simulink model "orangery_next_generation"  (R2020b)
settings: Solver=ode45  StartTime=86000*600  StopTime=86000*607  FixedStep=0.01  MaxStep=1  RelTol=1e-6  EnableMultiTasking=on
settings Model: Creator=oleg.kmechak  LastModifiedBy=ofcra
settings DataIOCC: LimitDataPoints=on  SaveFinalState=on  SaveFormat=Array  ReturnWorkspaceOutputs=off
settings OptimizationCC: LifeSpan=inf
settings DebuggingCC: UnderspecifiedInitializationDetection=Classic  MergeDetectMultiDrivingBlocksExec=none  SolverPrmCheckMsg=warning  SFUnexpectedBacktrackingDiag=warning  SFNoUnconditionalDefaultTransitionDiag=warning  SFExecutionAtInitializationDiag=none  ArithmeticOperatorsInVariantConditions=warning
settings HardwareCC: ProdBitPerPointer=32  ProdBitPerSizeT=32  ProdBitPerPtrDiffT=32  ProdLargestAtomicFloat=None  ProdIntDivRoundTo=Undefined  ProdEndianess=Unspecified  ProdWordSize=32  ProdHWDeviceType=32-bit Generic
settings ModelReferenceCC: PropagateSignalLabelsOutOfModel=off
settings SFSimCC: SimUseLocalCustomCode=off  CustomCodeUndefinedFunction=UseInterfaceOnly
settings RTWCC: GenerateReport=on  RTWUseLocalCustomCode=off  LaunchReport=on
settings CodeAppCC: ForceParamTrailComments=on  StateflowObjectComments=on  MATLABSourceComments=on
settings GRTTargetCC: TargetLangStandard=C89/C90 (ANSI)
settings ConfigComp: CovMetricSettings=dw  CovSaveCumulativeToWorkspaceVar=on  CovSaveSingleToWorkspaceVar=on  CovExternalEMLEnable=off

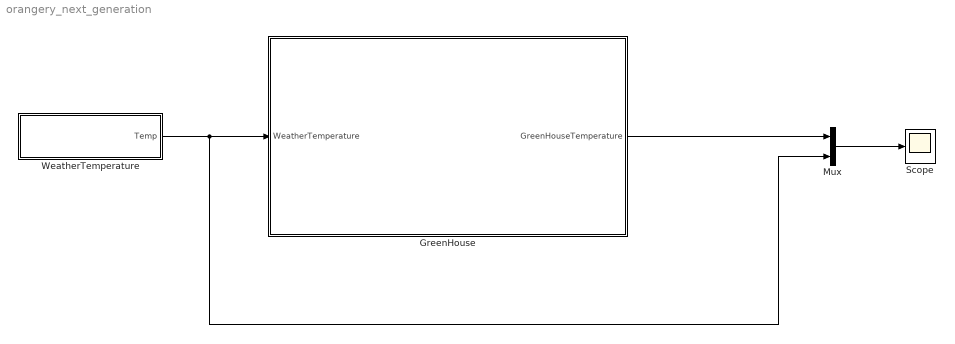
== system orangery_next_generation ==
  GreenHouse : Subsystem  mask{alpha=2.68, S=40, p=1.293, c=1006, V=53}
      mask prompts: alpha "thermal conductivity"; S "Square"; p "density"; V "Volume"
  Mux : Mux  Inputs=2
  Scope : Scope
  WeatherTemperature : Subsystem
  wires:
  WeatherTemperature/1(Temp) -> Mux/2, GreenHouse/1(WeatherTemperature)
  GreenHouse/1(GreenHouseTemperature) -> Mux/1
  Mux/1 -> Scope/1

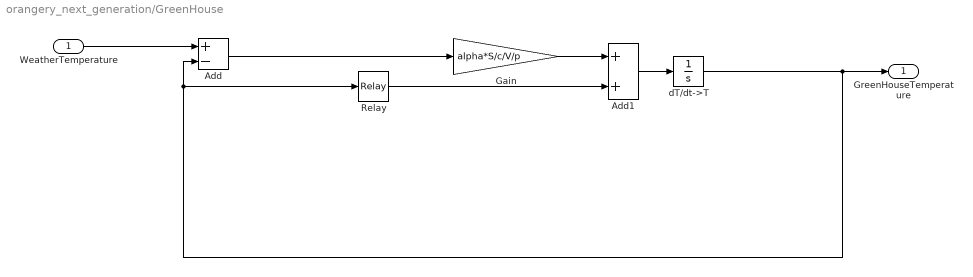
== system orangery_next_generation/GreenHouse ==
  WeatherTemperature : Inport
  Add : Sum  Inputs=+-
  Add1 : Sum
  Gain : Gain  Gain=alpha*S/c/V/p
  Relay : Relay  OnSwitchValue=268.5  OffSwitchValue=268  OnOutputValue=0  OffOutputValue=0.0001
  dT/dt->T : Integrator  InitialCondition=270
  GreenHouseTemperature : Outport
  wires:
  Add/1 -> Gain/1
  dT/dt->T/1 -> GreenHouseTemperature/1, Relay/1, Add/2
  WeatherTemperature/1 -> Add/1
  Add1/1 -> dT/dt->T/1
  Gain/1 -> Add1/1
  Relay/1 -> Add1/2

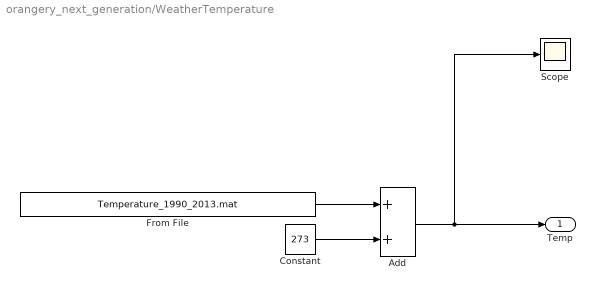
== system orangery_next_generation/WeatherTemperature ==
  Add : Sum
  Constant : Constant  Value=273
  From File : FromFile  FileName=Temperature_1990_2013.mat  SampleTime=0
  Scope : Scope
  Temp : Outport
  wires:
  Add/1 -> Scope/1, Temp/1
  Constant/1 -> Add/2
  From File/1 -> Add/1
